simulink model "IBR_Control_2024b"  (R2024b)
settings: Solver=ode4  StartTime=0.0  StopTime=1  FixedStep=Ts  RelTol=1e-3
values from neighbouring files (symbols this model uses):
  Fn = Simulink.Parameter    [IBR_Control_Parameters.m]
  Iang0_pcc = Simulink.Parameter    [IBR_Control_Parameters.m]
  Imag0_pcc = Simulink.Parameter    [IBR_Control_Parameters.m]
  Ki_I = Simulink.Parameter    [IBR_Control_Parameters.m]
  Ki_PLL = Simulink.Parameter    [IBR_Control_Parameters.m]
  Kp_I = Simulink.Parameter    [IBR_Control_Parameters.m]
  Kp_PLL = Simulink.Parameter    [IBR_Control_Parameters.m]
  Lc = Simulink.Parameter    [IBR_Control_Parameters.m]
  Pref = Simulink.Parameter    [IBR_Control_Parameters.m]
  Qref = Simulink.Parameter    [IBR_Control_Parameters.m]
  Rc = Simulink.Parameter    [IBR_Control_Parameters.m]
  Tf_S = Simulink.Parameter    [IBR_Control_Parameters.m]
  Ts = Simulink.Parameter    [IBR_Control_Parameters.m]
  Vang0_pcc = Simulink.Parameter    [IBR_Control_Parameters.m]
  Vmag0_pcc = Simulink.Parameter    [IBR_Control_Parameters.m]
undefined symbols (not defined in the file or in its folder): DiscIntNeverNeededParam
libraries: slpidlib x3, model_info x1
settings Model: ParamWorkspaceSource=ReferencedWorkspace  Creator=evansolingen  LastModifiedBy=if47izeq
settings DataIOCC: LimitDataPoints=on  SaveFormat=Array  SignalLoggingSaveFormat=ModelDataLogs  SaveOutput=off  SignalLogging=off  SaveTime=off  ReturnWorkspaceOutputs=off
settings OptimizationCC: EnhancedBackFolding=on  ExpressionFolding=off  PassReuseOutputArgsThreshold=0  ExpressionDepthLimit=2147483647  OptimizeBlockOrder=speed  DifferentSizesBufferReuse=on
settings DebuggingCC: UnderspecifiedInitializationDetection=Classic  MergeDetectMultiDrivingBlocksExec=none  SolverPrmCheckMsg=warning  MultiTaskDSMMsg=warning  MultiTaskCondExecSysMsg=none  ParameterTunabilityLossMsg=error  FcnCallInpInsideContextMsg=warning  UnconnectedInputMsg=warning  UnconnectedOutputMsg=warning  UnconnectedLineMsg=warning  AllowSymbolicDim=off  StateNameClashWarn=warning  SFUnexpectedBacktrackingDiag=warning  SFNoUnconditionalDefaultTransitionDiag=warning  SFExecutionAtInitializationDiag=none  ArithmeticOperatorsInVariantConditions=warning
settings HardwareCC: ProdBitPerPointer=32  ProdBitPerSizeT=32  ProdBitPerPtrDiffT=32  ProdLargestAtomicFloat=None  ProdIntDivRoundTo=Undefined  ProdEndianess=Unspecified  ProdWordSize=32  ProdHWDeviceType=32-bit Generic
settings ModelReferenceCC: UpdateModelReferenceTargets=Force  EnableRefExpFcnMdlSchedulingChecks=on  PropagateSignalLabelsOutOfModel=off
settings SFSimCC: SimUseLocalCustomCode=off  SimParseCustomCode=off  MATLABDynamicMemAlloc=off  CustomCodeUndefinedFunction=UseInterfaceOnly
settings RTWCC: Description=Create Visual C/C++ Solution File for Simulink Coder  SystemTargetFile=IEC61400_27_DLL.tlc  TemplateMakefile=IEC61400_27_DLL.tmf  RTWUseLocalCustomCode=off  GPUComputeCapability=3.5
settings CodeAppCC: ForceParamTrailComments=on  OperatorAnnotations=on
settings STFCustomTargetCC: ModelReferenceCompliant=off  MATLABClassNameForMDSCustomization=Simulink.SoftwareTarget.TargetSpecificTriggerConfigurationBase  GRTInterface=on  SystemTargetFile=IEC61400_27_DLL.tlc
settings ConfigComp: CovMetricSettings=dw  CovSaveCumulativeToWorkspaceVar=on  CovSaveSingleToWorkspaceVar=on  CovExternalEMLEnable=off

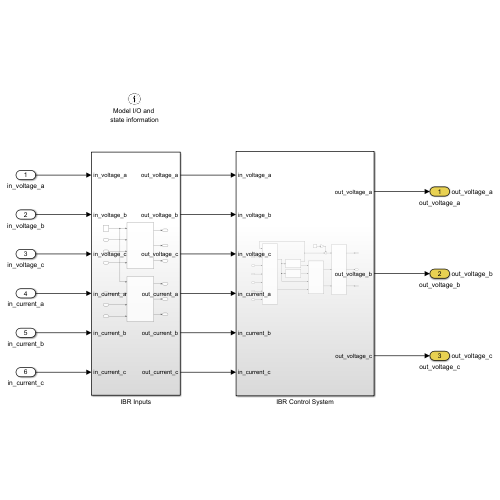
[thumbnail: Simulink's stored preview of the top-level diagram]
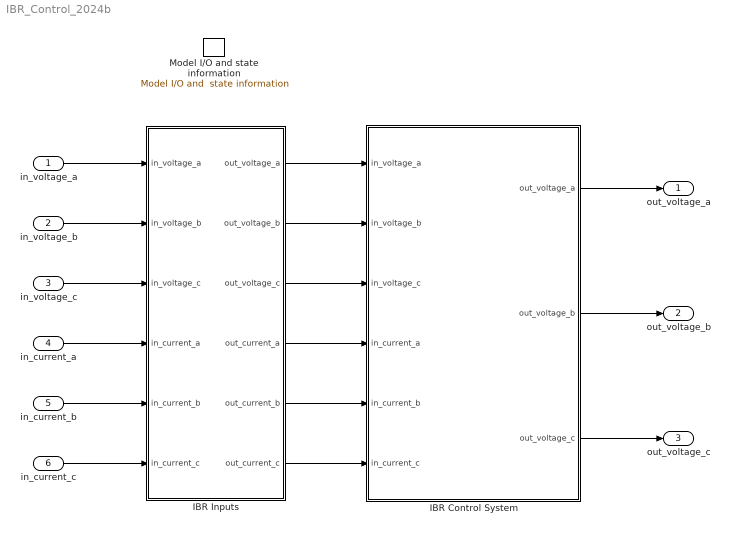
== system IBR_Control_2024b ==
  in_voltage_a : Inport
  in_voltage_b : Inport  Port=2
  in_voltage_c : Inport  Port=3
  in_current_a : Inport  Port=4
  in_current_b : Inport  Port=5
  in_current_c : Inport  Port=6
  IBR Control System : Subsystem
  IBR Inputs : Subsystem
  Model I/O and state information : model_info/Model I//O and  state information
  out_voltage_a : Outport  SignalName=out_voltage_a
  out_voltage_b : Outport  Port=2  SignalName=out_voltage_b
  out_voltage_c : Outport  Port=3  SignalName=out_voltage_c
  wires:
  IBR Control System/1(out_voltage_a) -> out_voltage_a/1
  IBR Control System/2(out_voltage_b) -> out_voltage_b/1
  IBR Control System/3(out_voltage_c) -> out_voltage_c/1
  in_voltage_a/1 -> IBR Inputs/1(in_voltage_a)
  in_voltage_b/1 -> IBR Inputs/2(in_voltage_b)
  in_voltage_c/1 -> IBR Inputs/3(in_voltage_c)
  in_current_a/1 -> IBR Inputs/4(in_current_a)
  in_current_b/1 -> IBR Inputs/5(in_current_b)
  in_current_c/1 -> IBR Inputs/6(in_current_c)
  IBR Inputs/1(out_voltage_a) -> IBR Control System/1(in_voltage_a)
  IBR Inputs/2(out_voltage_b) -> IBR Control System/2(in_voltage_b)
  IBR Inputs/3(out_voltage_c) -> IBR Control System/3(in_voltage_c)
  IBR Inputs/4(out_current_a) -> IBR Control System/4(in_current_a)
  IBR Inputs/6(out_current_c) -> IBR Control System/6(in_current_c)
  IBR Inputs/5(out_current_b) -> IBR Control System/5(in_current_b)

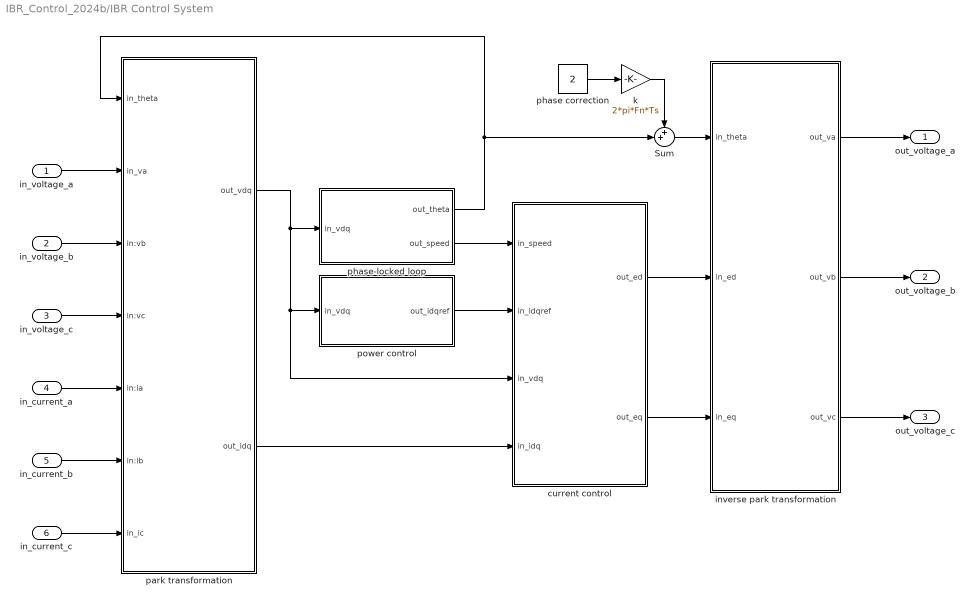
== system IBR_Control_2024b/IBR Control System ==
  in_voltage_a : Inport
  in_voltage_b : Inport  Port=2
  in_voltage_c : Inport  Port=3
  in_current_a : Inport  Port=4
  in_current_b : Inport  Port=5
  in_current_c : Inport  Port=6
  Sum : Sum  Inputs=++|
  current control : Subsystem
  inverse park transformation : Subsystem
  k : Gain  Gain=2*pi*Fn*Ts
  park transformation : Subsystem
  phase correction : Constant  Value=2
  phase-locked loop : Subsystem
  power control : Subsystem
  out_voltage_a : Outport
  out_voltage_b : Outport  Port=2
  out_voltage_c : Outport  Port=3
  wires:
  in_current_b/1 -> park transformation/6(in:ib)
  in_current_c/1 -> park transformation/7(in_ic)
  in_current_a/1 -> park transformation/5(in:ia)
  in_voltage_a/1 -> park transformation/2(in_va)
  in_voltage_b/1 -> park transformation/3(in:vb)
  in_voltage_c/1 -> park transformation/4(in:vc)
  park transformation/1(out_vdq) -> current control/3(in_vdq), power control/1(in_vdq), phase-locked loop/1(in_vdq)
  park transformation/2(out_idq) -> current control/4(in_idq)
  phase-locked loop/2(out_speed) -> current control/1(in_speed)
  power control/1(out_idqref) -> current control/2(in_idqref)
  inverse park transformation/1(out_va) -> out_voltage_a/1
  inverse park transformation/2(out_vb) -> out_voltage_b/1
  inverse park transformation/3(out_vc) -> out_voltage_c/1
  current control/1(out_ed) -> inverse park transformation/2(in_ed)
  current control/2(out_eq) -> inverse park transformation/3(in_eq)
  Sum/1 -> inverse park transformation/1(in_theta)
  phase-locked loop/1(out_theta) -> Sum/2, park transformation/1(in_theta)
  phase correction/1 -> k/1
  k/1 -> Sum/1

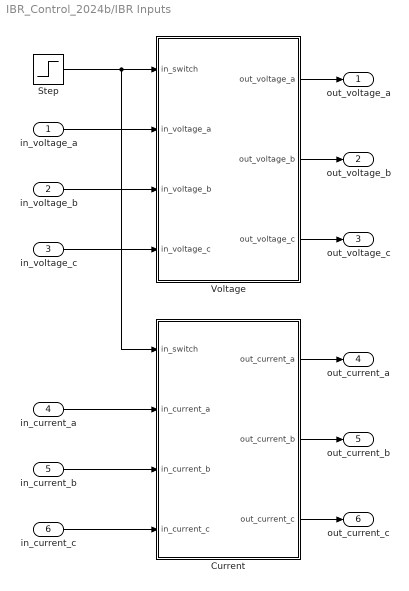
== system IBR_Control_2024b/IBR Inputs ==
  in_voltage_a : Inport
  in_voltage_b : Inport  Port=2
  in_voltage_c : Inport  Port=3
  in_current_a : Inport  Port=4
  in_current_b : Inport  Port=5
  in_current_c : Inport  Port=6
  Current : Subsystem
  Step : Step  Time=3*Ts  Before=1  After=0  SampleTime=0
  Voltage : Subsystem
  out_voltage_a : Outport
  out_voltage_b : Outport  Port=2
  out_voltage_c : Outport  Port=3
  out_current_a : Outport  Port=4
  out_current_b : Outport  Port=5
  out_current_c : Outport  Port=6
  wires:
  Step/1 -> Voltage/1(in_switch), Current/1(in_switch)
  in_voltage_a/1 -> Voltage/2(in_voltage_a)
  in_voltage_c/1 -> Voltage/4(in_voltage_c)
  Voltage/1(out_voltage_a) -> out_voltage_a/1
  Voltage/2(out_voltage_b) -> out_voltage_b/1
  Voltage/3(out_voltage_c) -> out_voltage_c/1
  in_voltage_b/1 -> Voltage/3(in_voltage_b)
  in_current_a/1 -> Current/2(in_current_a)
  in_current_b/1 -> Current/3(in_current_b)
  in_current_c/1 -> Current/4(in_current_c)
  Current/1(out_current_a) -> out_current_a/1
  Current/2(out_current_b) -> out_current_b/1
  Current/3(out_current_c) -> out_current_c/1

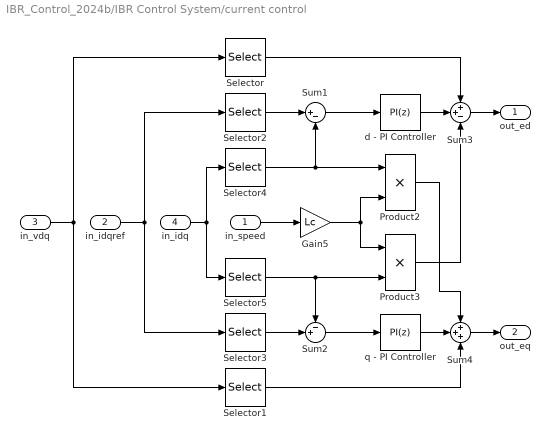
== system IBR_Control_2024b/IBR Control System/current control ==
  in_speed : Inport
  in_idqref : Inport  Port=2
  in_vdq : Inport  Port=3
  in_idq : Inport  Port=4
  Gain5 : Gain  Gain=Lc
  Product2 : Product
  Product3 : Product
  Selector : Selector  InputPortWidth=2  IndexOptions=Index vector (dialog)  Indices=1  OutputSizes=1
  Selector1 : Selector  InputPortWidth=2  IndexOptions=Index vector (dialog)  Indices=[2]  OutputSizes=1
  Selector2 : Selector  InputPortWidth=2  IndexOptions=Index vector (dialog)  Indices=[1]  OutputSizes=1
  Selector3 : Selector  InputPortWidth=2  IndexOptions=Index vector (dialog)  Indices=[2]  OutputSizes=1
  Selector4 : Selector  InputPortWidth=2  IndexOptions=Index vector (dialog)  Indices=[1]  OutputSizes=1
  Selector5 : Selector  InputPortWidth=2  IndexOptions=Index vector (dialog)  Indices=[2]  OutputSizes=1
  Sum1 : Sum  Inputs=|+-
  Sum2 : Sum  Inputs=-+|
  Sum3 : Sum  Inputs=++-
  Sum4 : Sum  Inputs=+++
  d - PI Controller : slpidlib/PID Controller  Controller=PI  Form=Parallel  TimeDomain=Discrete-time  UseExternalTs=off  SampleTime=-1  IntegratorMethod=Forward Euler  FilterMethod=Forward Euler  ControllerParametersSource=internal  P=Kp_I  I=Ki_I  UseKiTs=off  D=0  UseExternalDerivativeSource=off  N=100  UseFilter=on  TunerSelectOption=Transfer Function Based (PID Tuner App)  InitialConditionSource=internal  InitialConditionForIntegrator=Pref/(sqrt(3)/sqrt(2)*Vmag0_pcc)*Rc  InitialConditionForFilter=0  DifferentiatorICPrevScaledInput=0  ExternalReset=none  TrackingMode=off  Kt=1  LimitOutput=off  SatLimitsSource=internal  UpperSaturationLimit=inf  LowerSaturationLimit=-inf  LinearizeAsGain=on  AntiWindupMode=none  Kb=1  LimitIntegrator=off  UpperIntegratorSaturationLimit=inf  LowerIntegratorSaturationLimit=-inf  POutMin=[]  POutMax=[]  IOutMin=[]  IOutMax=[]  DOutMin=[]  DOutMax=[]  NOutMin=[]  NOutMax=[]  SumOutMin=[]  SumOutMax=[]  SaturationOutMin=[]  SaturationOutMax=[]  PParamMin=[]  PParamMax=[]  IParamMin=[]  IParamMax=[]  DParamMin=[]  DParamMax=[]  NParamMin=[]  NParamMax=[]  KbParamMin=[]  KbParamMax=[]  KtParamMin=[]  KtParamMax=[]  KbOutMin=[]  KbOutMax=[]  KtOutMin=[]  KtOutMax=[]  IntegratorOutMin=[]  IntegratorOutMax=[]  FilterOutMin=[]  FilterOutMax=[]  SumI1OutMin=[]  SumI1OutMax=[]  SumI2OutMin=[]  SumI2OutMax=[]  SumI3OutMin=[]  SumI3OutMax=[]  SumI4OutMin=[]  SumI4OutMax=[]  SumDOutMin=[]  SumDOutMax=[]  DifferentiatorOutMin=[]  DifferentiatorOutMax=[]  FilterDiffOutCoefMin=[]  FilterDiffOutCoefMax=[]  ReciprocalOutMin=[]  ReciprocalOutMax=[]  SumDenOutMin=[]  SumDenOutMax=[]  SumNumOutMin=[]  SumNumOutMax=[]  DivideOutMin=[]  DivideOutMax=[]  UdiffTsProdOutMin=[]  UdiffTsProdOutMax=[]  NTsProdOutMin=[]  NTsProdOutMax=[]  UintegralTsProdOutMin=[]  UintegralTsProdOutMax=[]  UngainTsProdOutMin=[]  UngainTsProdOutMax=[]  ClampingZeroOutDataTypeStr=Inherit: Inherit via back propagation  ClampingZeroOutMin=[]  ClampingZeroOutMax=[]  FilterDenConstantOutDataTypeStr=Inherit: Inherit via back propagation  FilterDenConstantOutMin=[]  FilterDenConstantOutMax=[]  PCopyOutDataTypeStr=Inherit: Inherit via back propagation  PCopyOutMin=[]  PCopyOutMax=[]  NCopyOutDataTypeStr=Inherit: Inherit via back propagation  NCopyOutMin=[]  NCopyOutMax=[]  IntegratorContinuousStateAttributes=''  IntegratorStateMustResolveToSignalObject=off  IntegratorRTWStateStorageClass=Auto  FilterContinuousStateAttributes=''  FilterStateMustResolveToSignalObject=off  FilterRTWStateStorageClass=Auto  ParallelPVariant=InternalParameters  IdealPVariant=Disabled  IVariant=InternalParameters  DVariant=Disabled  IntegratorVariant=Discrete  SatVariant=Disabled  AWVariant=Passthrough  PCopyVariant=Disabled  TRVariant=Disabled  FdbkBlocksVariant=Forward  IdealPFdbkVariant=Disabled  SatFdbkVariant=Disabled  DerivativeFilterVariant=Disabled  NVariant=Disabled  NCopyVariant=Disabled_SignalSpec  FilterICVariant=Disabled  IntegratorICVariant=InternalICs  ExternalResetVariant=Disabled  TRSumVariant=Passthrough  SumFdbkVariant=Disabled  SumVariant=Sum_PI  TsampFilterVariant=InternalTs  TsampNgainVariant=Passthrough  TsampIntegralVariant=Disabled_SignalSpec  ExternalSaturationOutDataTypeStr=Inherit: Same as second input  DerivativeSourceVariant=Disabled  PreIntVariant=InternalPreInt
  q - PI Controller : slpidlib/PID Controller  Controller=PI  Form=Parallel  TimeDomain=Discrete-time  UseExternalTs=off  SampleTime=-1  IntegratorMethod=Forward Euler  FilterMethod=Forward Euler  ControllerParametersSource=internal  P=Kp_I  I=Ki_I  UseKiTs=off  D=0  UseExternalDerivativeSource=off  N=100  UseFilter=on  TunerSelectOption=Transfer Function Based (PID Tuner App)  InitialConditionSource=internal  InitialConditionForIntegrator=-Qref/(sqrt(3)/sqrt(2)*Vmag0_pcc)*Rc  InitialConditionForFilter=0  DifferentiatorICPrevScaledInput=0  ExternalReset=none  TrackingMode=off  Kt=1  LimitOutput=off  SatLimitsSource=internal  UpperSaturationLimit=inf  LowerSaturationLimit=-inf  LinearizeAsGain=on  AntiWindupMode=none  Kb=1  LimitIntegrator=off  UpperIntegratorSaturationLimit=inf  LowerIntegratorSaturationLimit=-inf  POutMin=[]  POutMax=[]  IOutMin=[]  IOutMax=[]  DOutMin=[]  DOutMax=[]  NOutMin=[]  NOutMax=[]  SumOutMin=[]  SumOutMax=[]  SaturationOutMin=[]  SaturationOutMax=[]  PParamMin=[]  PParamMax=[]  IParamMin=[]  IParamMax=[]  DParamMin=[]  DParamMax=[]  NParamMin=[]  NParamMax=[]  KbParamMin=[]  KbParamMax=[]  KtParamMin=[]  KtParamMax=[]  KbOutMin=[]  KbOutMax=[]  KtOutMin=[]  KtOutMax=[]  IntegratorOutMin=[]  IntegratorOutMax=[]  FilterOutMin=[]  FilterOutMax=[]  SumI1OutMin=[]  SumI1OutMax=[]  SumI2OutMin=[]  SumI2OutMax=[]  SumI3OutMin=[]  SumI3OutMax=[]  SumI4OutMin=[]  SumI4OutMax=[]  SumDOutMin=[]  SumDOutMax=[]  DifferentiatorOutMin=[]  DifferentiatorOutMax=[]  FilterDiffOutCoefMin=[]  FilterDiffOutCoefMax=[]  ReciprocalOutMin=[]  ReciprocalOutMax=[]  SumDenOutMin=[]  SumDenOutMax=[]  SumNumOutMin=[]  SumNumOutMax=[]  DivideOutMin=[]  DivideOutMax=[]  UdiffTsProdOutMin=[]  UdiffTsProdOutMax=[]  NTsProdOutMin=[]  NTsProdOutMax=[]  UintegralTsProdOutMin=[]  UintegralTsProdOutMax=[]  UngainTsProdOutMin=[]  UngainTsProdOutMax=[]  ClampingZeroOutDataTypeStr=Inherit: Inherit via back propagation  ClampingZeroOutMin=[]  ClampingZeroOutMax=[]  FilterDenConstantOutDataTypeStr=Inherit: Inherit via back propagation  FilterDenConstantOutMin=[]  FilterDenConstantOutMax=[]  PCopyOutDataTypeStr=Inherit: Inherit via back propagation  PCopyOutMin=[]  PCopyOutMax=[]  NCopyOutDataTypeStr=Inherit: Inherit via back propagation  NCopyOutMin=[]  NCopyOutMax=[]  IntegratorContinuousStateAttributes=''  IntegratorStateMustResolveToSignalObject=off  IntegratorRTWStateStorageClass=Auto  FilterContinuousStateAttributes=''  FilterStateMustResolveToSignalObject=off  FilterRTWStateStorageClass=Auto  ParallelPVariant=InternalParameters  IdealPVariant=Disabled  IVariant=InternalParameters  DVariant=Disabled  IntegratorVariant=Discrete  SatVariant=Disabled  AWVariant=Passthrough  PCopyVariant=Disabled  TRVariant=Disabled  FdbkBlocksVariant=Forward  IdealPFdbkVariant=Disabled  SatFdbkVariant=Disabled  DerivativeFilterVariant=Disabled  NVariant=Disabled  NCopyVariant=Disabled_SignalSpec  FilterICVariant=Disabled  IntegratorICVariant=InternalICs  ExternalResetVariant=Disabled  TRSumVariant=Passthrough  SumFdbkVariant=Disabled  SumVariant=Sum_PI  TsampFilterVariant=InternalTs  TsampNgainVariant=Passthrough  TsampIntegralVariant=Disabled_SignalSpec  ExternalSaturationOutDataTypeStr=Inherit: Same as second input  DerivativeSourceVariant=Disabled  PreIntVariant=InternalPreInt
  out_ed : Outport
  out_eq : Outport  Port=2
  wires:
  Gain5/1 -> Product2/2, Product3/1
  Sum4/1 -> out_eq/1
  Product3/1 -> Sum3/3
  Selector3/1 -> Sum2/2
  Sum1/1 -> d - PI Controller/1
  Sum3/1 -> out_ed/1
  Product2/1 -> Sum4/1
  Sum2/1 -> q - PI Controller/1
  in_speed/1 -> Gain5/1
  in_vdq/1 -> Selector1/1, Selector/1
  in_idq/1 -> Selector5/1, Selector4/1
  Selector5/1 -> Product3/2, Sum2/1
  d - PI Controller/1 -> Sum3/2
  q - PI Controller/1 -> Sum4/2
  Selector1/1 -> Sum4/3
  in_idqref/1 -> Selector2/1, Selector3/1
  Selector2/1 -> Sum1/1
  Selector/1 -> Sum3/1
  Selector4/1 -> Product2/1, Sum1/2

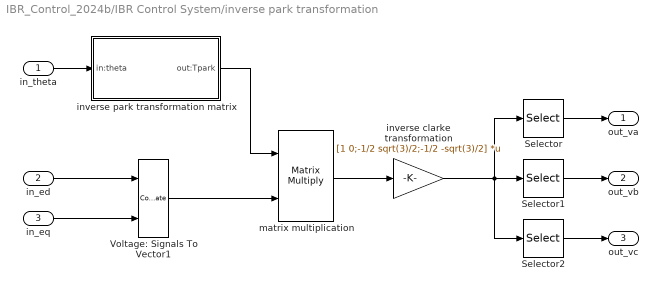
== system IBR_Control_2024b/IBR Control System/inverse park transformation ==
  in_theta : Inport
  in_ed : Inport  Port=2
  in_eq : Inport  Port=3
  Selector : Selector  InputPortWidth=3  IndexOptions=Index vector (dialog)  Indices=[1]  OutputSizes=1
  Selector1 : Selector  InputPortWidth=3  IndexOptions=Index vector (dialog)  Indices=[2]  OutputSizes=1
  Selector2 : Selector  InputPortWidth=3  IndexOptions=Index vector (dialog)  Indices=[3]  OutputSizes=1
  Voltage: Signals To Vector1 : Concatenate  Mode=Multidimensional array
  inverse clarke transformation : Gain  Gain=[1 0;-1/2 sqrt(3)/2;-1/2 -sqrt(3)/2]  Multiplication=Matrix(K*u)
  inverse park transformation matrix : Subsystem
  matrix multiplication : Product  Multiplication=Matrix(*)
  out_va : Outport
  out_vb : Outport  Port=2
  out_vc : Outport  Port=3
  wires:
  inverse park transformation matrix/1(out:Tpark) -> matrix multiplication/1
  in_theta/1 -> inverse park transformation matrix/1(in:theta)
  inverse clarke transformation/1 -> Selector2/1, Selector1/1, Selector/1
  matrix multiplication/1 -> inverse clarke transformation/1
  Selector1/1 -> out_vb/1
  Selector/1 -> out_va/1
  in_ed/1 -> Voltage: Signals To Vector1/1
  in_eq/1 -> Voltage: Signals To Vector1/2
  Voltage: Signals To Vector1/1 -> matrix multiplication/2
  Selector2/1 -> out_vc/1

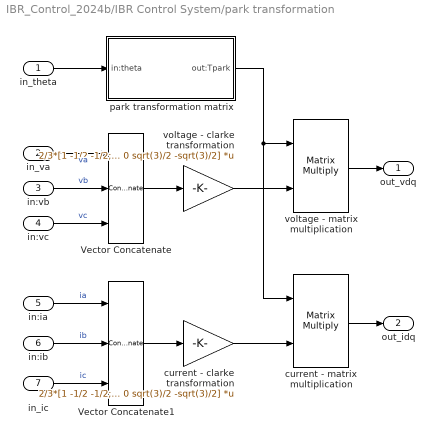
== system IBR_Control_2024b/IBR Control System/park transformation ==
  in_theta : Inport
  in_va : Inport  Port=2
  in:vb : Inport  Port=3
  in:vc : Inport  Port=4
  in:ia : Inport  Port=5
  in:ib : Inport  Port=6
  in_ic : Inport  Port=7
  Vector Concatenate : Concatenate  NumInputs=3  Mode=Multidimensional array
  Vector Concatenate1 : Concatenate  NumInputs=3  Mode=Multidimensional array
  current - clarke transformation : Gain  Gain=2/3*[1 -1/2 -1/2; 0 sqrt(3)/2 -sqrt(3)/2]  Multiplication=Matrix(K*u)
  current - matrix multiplication : Product  Multiplication=Matrix(*)
  park transformation matrix : Subsystem
  voltage - clarke transformation : Gain  Gain=2/3*[1 -1/2 -1/2; 0 sqrt(3)/2 -sqrt(3)/2]  Multiplication=Matrix(K*u)
  voltage - matrix multiplication : Product  Multiplication=Matrix(*)
  out_vdq : Outport
  out_idq : Outport  Port=2
  wires:
  in_va/1 -> Vector Concatenate/1  "va"
  in:ib/1 -> Vector Concatenate1/2  "ib"
  in_ic/1 -> Vector Concatenate1/3  "ic"
  Vector Concatenate1/1 -> current - clarke transformation/1
  in:ia/1 -> Vector Concatenate1/1  "ia"
  voltage - matrix multiplication/1 -> out_vdq/1
  in:vb/1 -> Vector Concatenate/2  "vb"
  in:vc/1 -> Vector Concatenate/3  "vc"
  Vector Concatenate/1 -> voltage - clarke transformation/1
  voltage - clarke transformation/1 -> voltage - matrix multiplication/2
  current - clarke transformation/1 -> current - matrix multiplication/2
  park transformation matrix/1(out:Tpark) -> voltage - matrix multiplication/1, current - matrix multiplication/1
  current - matrix multiplication/1 -> out_idq/1
  in_theta/1 -> park transformation matrix/1(in:theta)

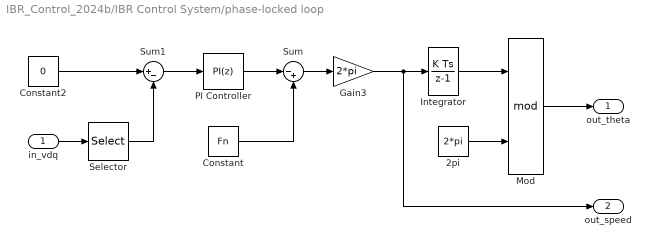
== system IBR_Control_2024b/IBR Control System/phase-locked loop ==
  in_vdq : Inport
  2pi : Constant  Value=2*pi
  Constant : Constant  Value=Fn
  Constant2 : Constant  Value=0
  Gain3 : Gain  Gain=2*pi
  Integrator : DiscreteIntegrator  InitialCondition=Vang0_pcc-2*2*pi*Fn*Ts  SampleTime=-1  ICPrevOutput=DiscIntNeverNeededParam  ICPrevScaledInput=DiscIntNeverNeededParam
  Mod : Math  Operator=mod
  PI Controller : slpidlib/PID Controller  Controller=PI  Form=Parallel  TimeDomain=Discrete-time  UseExternalTs=off  SampleTime=-1  IntegratorMethod=Forward Euler  FilterMethod=Forward Euler  ControllerParametersSource=internal  P=Kp_PLL  I=Ki_PLL  UseKiTs=off  D=0  UseExternalDerivativeSource=off  N=100  UseFilter=on  TunerSelectOption=Transfer Function Based (PID Tuner App)  InitialConditionSource=internal  InitialConditionForIntegrator=0  InitialConditionForFilter=0  DifferentiatorICPrevScaledInput=0  ExternalReset=none  TrackingMode=off  Kt=1  LimitOutput=off  SatLimitsSource=internal  UpperSaturationLimit=inf  LowerSaturationLimit=-inf  LinearizeAsGain=on  AntiWindupMode=none  Kb=1  LimitIntegrator=off  UpperIntegratorSaturationLimit=inf  LowerIntegratorSaturationLimit=-inf  POutMin=[]  POutMax=[]  IOutMin=[]  IOutMax=[]  DOutMin=[]  DOutMax=[]  NOutMin=[]  NOutMax=[]  SumOutMin=[]  SumOutMax=[]  SaturationOutMin=[]  SaturationOutMax=[]  PParamMin=[]  PParamMax=[]  IParamMin=[]  IParamMax=[]  DParamMin=[]  DParamMax=[]  NParamMin=[]  NParamMax=[]  KbParamMin=[]  KbParamMax=[]  KtParamMin=[]  KtParamMax=[]  KbOutMin=[]  KbOutMax=[]  KtOutMin=[]  KtOutMax=[]  IntegratorOutMin=[]  IntegratorOutMax=[]  FilterOutMin=[]  FilterOutMax=[]  SumI1OutMin=[]  SumI1OutMax=[]  SumI2OutMin=[]  SumI2OutMax=[]  SumI3OutMin=[]  SumI3OutMax=[]  SumI4OutMin=[]  SumI4OutMax=[]  SumDOutMin=[]  SumDOutMax=[]  DifferentiatorOutMin=[]  DifferentiatorOutMax=[]  FilterDiffOutCoefMin=[]  FilterDiffOutCoefMax=[]  ReciprocalOutMin=[]  ReciprocalOutMax=[]  SumDenOutMin=[]  SumDenOutMax=[]  SumNumOutMin=[]  SumNumOutMax=[]  DivideOutMin=[]  DivideOutMax=[]  UdiffTsProdOutMin=[]  UdiffTsProdOutMax=[]  NTsProdOutMin=[]  NTsProdOutMax=[]  UintegralTsProdOutMin=[]  UintegralTsProdOutMax=[]  UngainTsProdOutMin=[]  UngainTsProdOutMax=[]  ClampingZeroOutDataTypeStr=Inherit: Inherit via back propagation  ClampingZeroOutMin=[]  ClampingZeroOutMax=[]  FilterDenConstantOutDataTypeStr=Inherit: Inherit via back propagation  FilterDenConstantOutMin=[]  FilterDenConstantOutMax=[]  PCopyOutDataTypeStr=Inherit: Inherit via back propagation  PCopyOutMin=[]  PCopyOutMax=[]  NCopyOutDataTypeStr=Inherit: Inherit via back propagation  NCopyOutMin=[]  NCopyOutMax=[]  IntegratorContinuousStateAttributes=''  IntegratorStateMustResolveToSignalObject=off  IntegratorRTWStateStorageClass=Auto  FilterContinuousStateAttributes=''  FilterStateMustResolveToSignalObject=off  FilterRTWStateStorageClass=Auto  ParallelPVariant=InternalParameters  IdealPVariant=Disabled  IVariant=InternalParameters  DVariant=Disabled  IntegratorVariant=Discrete  SatVariant=Disabled  AWVariant=Passthrough  PCopyVariant=Disabled  TRVariant=Disabled  FdbkBlocksVariant=Forward  IdealPFdbkVariant=Disabled  SatFdbkVariant=Disabled  DerivativeFilterVariant=Disabled  NVariant=Disabled  NCopyVariant=Disabled_SignalSpec  FilterICVariant=Disabled  IntegratorICVariant=InternalICs  ExternalResetVariant=Disabled  TRSumVariant=Passthrough  SumFdbkVariant=Disabled  SumVariant=Sum_PI  TsampFilterVariant=InternalTs  TsampNgainVariant=Passthrough  TsampIntegralVariant=Disabled_SignalSpec  ExternalSaturationOutDataTypeStr=Inherit: Same as second input  DerivativeSourceVariant=Disabled  PreIntVariant=InternalPreInt
  Selector : Selector  InputPortWidth=2  IndexOptions=Index vector (dialog)  Indices=[2]  OutputSizes=1
  Sum : Sum  Inputs=|-+
  Sum1 : Sum  Inputs=|+-
  out_theta : Outport
  out_speed : Outport  Port=2
  wires:
  Constant/1 -> Sum/2
  Sum/1 -> Gain3/1
  2pi/1 -> Mod/2
  Gain3/1 -> out_speed/1, Integrator/1
  Sum1/1 -> PI Controller/1
  Mod/1 -> out_theta/1
  in_vdq/1 -> Selector/1
  Selector/1 -> Sum1/2
  Constant2/1 -> Sum1/1
  PI Controller/1 -> Sum/1
  Integrator/1 -> Mod/1

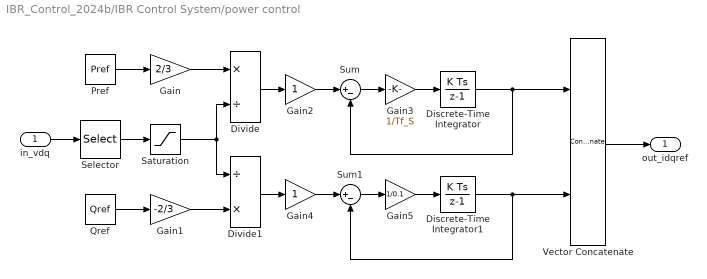
== system IBR_Control_2024b/IBR Control System/power control ==
  in_vdq : Inport
  Discrete-Time Integrator : DiscreteIntegrator  InitialCondition=Pref/(sqrt(3)/sqrt(2)*Vmag0_pcc)  SampleTime=-1  ICPrevOutput=DiscIntNeverNeededParam  ICPrevScaledInput=DiscIntNeverNeededParam
  Discrete-Time Integrator1 : DiscreteIntegrator  InitialCondition=-Qref/(sqrt(3)/sqrt(2)*Vmag0_pcc)  SampleTime=-1  ICPrevOutput=DiscIntNeverNeededParam  ICPrevScaledInput=DiscIntNeverNeededParam
  Divide : Product  Inputs=*/
  Divide1 : Product  Inputs=/*
  Gain : Gain  Gain=2/3
  Gain1 : Gain  Gain=-2/3
  Gain2 : Gain
  Gain3 : Gain  Gain=1/Tf_S
  Gain4 : Gain
  Gain5 : Gain  Gain=1/0.1
  Pref : Constant  Value=Pref
  Qref : Constant  Value=Qref
  Saturation : Saturate  UpperLimit=inf  LowerLimit=0.1
  Selector : Selector  InputPortWidth=2  IndexOptions=Index vector (dialog)  Indices=[1]  OutputSizes=1
  Sum : Sum  Inputs=|+-
  Sum1 : Sum  Inputs=|+-
  Vector Concatenate : Concatenate  Mode=Multidimensional array
  out_idqref : Outport
  wires:
  Pref/1 -> Gain/1
  Gain/1 -> Divide/1
  Qref/1 -> Gain1/1
  Selector/1 -> Saturation/1
  Gain1/1 -> Divide1/2
  in_vdq/1 -> Selector/1
  Vector Concatenate/1 -> out_idqref/1
  Divide/1 -> Gain2/1
  Gain2/1 -> Sum/1
  Sum/1 -> Gain3/1
  Gain3/1 -> Discrete-Time Integrator/1
  Discrete-Time Integrator/1 -> Sum/2, Vector Concatenate/1
  Sum1/1 -> Gain5/1
  Gain4/1 -> Sum1/1
  Gain5/1 -> Discrete-Time Integrator1/1
  Discrete-Time Integrator1/1 -> Vector Concatenate/2, Sum1/2
  Divide1/1 -> Gain4/1
  Saturation/1 -> Divide/2, Divide1/1

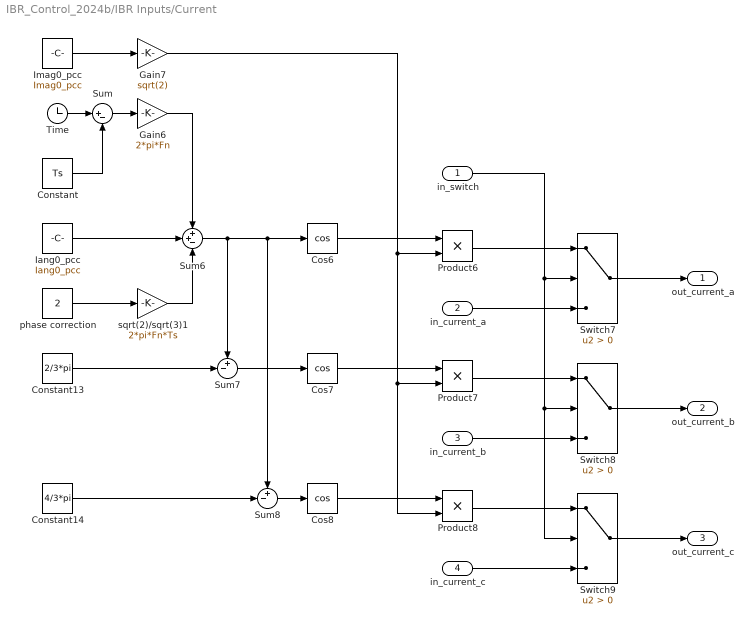
== system IBR_Control_2024b/IBR Inputs/Current ==
  in_switch : Inport
  in_current_a : Inport  Port=2
  in_current_b : Inport  Port=3
  in_current_c : Inport  Port=4
  Constant : Constant  Value=Ts
  Constant13 : Constant  Value=2/3*pi
  Constant14 : Constant  Value=4/3*pi
  Cos6 : Trigonometry  Operator=cos
  Cos7 : Trigonometry  Operator=cos
  Cos8 : Trigonometry  Operator=cos
  Gain6 : Gain  Gain=2*pi*Fn
  Gain7 : Gain  Gain=sqrt(2)
  Iang0_pcc : Constant  Value=Iang0_pcc
  Imag0_pcc : Constant  Value=Imag0_pcc
  Product6 : Product
  Product7 : Product
  Product8 : Product
  Sum : Sum  Inputs=|+-
  Sum6 : Sum  Inputs=++-
  Sum7 : Sum  Inputs=+-|
  Sum8 : Sum  Inputs=+-|
  Switch7 : Switch  Criteria=u2 > Threshold  SaturateOnIntegerOverflow=off  InputSameDT=off
  Switch8 : Switch  Criteria=u2 > Threshold  SaturateOnIntegerOverflow=off  InputSameDT=off
  Switch9 : Switch  Criteria=u2 > Threshold  SaturateOnIntegerOverflow=off  InputSameDT=off
  Time : Clock
  phase correction : Constant  Value=2
  sqrt(2)/sqrt(3)1 : Gain  Gain=2*pi*Fn*Ts
  out_current_a : Outport
  out_current_b : Outport  Port=2
  out_current_c : Outport  Port=3
  wires:
  Sum8/1 -> Cos8/1
  Gain7/1 -> Product8/2, Product7/2, Product6/2
  Cos7/1 -> Product7/1
  Switch9/1 -> out_current_c/1
  Constant14/1 -> Sum8/2
  Sum6/1 -> Cos6/1, Sum8/1, Sum7/1
  in_switch/1 -> Switch8/2, Switch9/2, Switch7/2
  Cos8/1 -> Product8/1
  Cos6/1 -> Product6/1
  Switch7/1 -> out_current_a/1
  Sum7/1 -> Cos7/1
  Iang0_pcc/1 -> Sum6/2
  Imag0_pcc/1 -> Gain7/1
  Product6/1 -> Switch7/1
  in_current_a/1 -> Switch7/3
  in_current_c/1 -> Switch9/3
  Product8/1 -> Switch9/1
  Product7/1 -> Switch8/1
  Constant13/1 -> Sum7/2
  Time/1 -> Sum/1
  Switch8/1 -> out_current_b/1
  in_current_b/1 -> Switch8/3
  phase correction/1 -> sqrt(2)/sqrt(3)1/1
  Gain6/1 -> Sum6/1
  sqrt(2)/sqrt(3)1/1 -> Sum6/3
  Constant/1 -> Sum/2
  Sum/1 -> Gain6/1

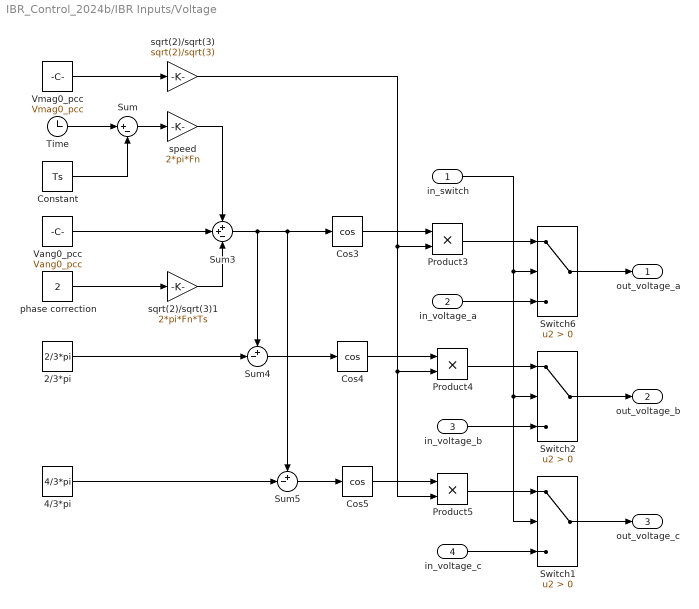
== system IBR_Control_2024b/IBR Inputs/Voltage ==
  in_switch : Inport
  in_voltage_a : Inport  Port=2
  in_voltage_b : Inport  Port=3
  in_voltage_c : Inport  Port=4
  2/3*pi : Constant  Value=2/3*pi
  4/3*pi : Constant  Value=4/3*pi
  Constant : Constant  Value=Ts
  Cos3 : Trigonometry  Operator=cos
  Cos4 : Trigonometry  Operator=cos
  Cos5 : Trigonometry  Operator=cos
  Product3 : Product
  Product4 : Product
  Product5 : Product
  Sum : Sum  Inputs=|+-
  Sum3 : Sum  Inputs=++-
  Sum4 : Sum  Inputs=+-|
  Sum5 : Sum  Inputs=+-|
  Switch1 : Switch  Criteria=u2 > Threshold  SaturateOnIntegerOverflow=off  InputSameDT=off
  Switch2 : Switch  Criteria=u2 > Threshold  SaturateOnIntegerOverflow=off  InputSameDT=off
  Switch6 : Switch  Criteria=u2 > Threshold  SaturateOnIntegerOverflow=off  InputSameDT=off
  Time : Clock
  Vang0_pcc : Constant  Value=Vang0_pcc
  Vmag0_pcc : Constant  Value=Vmag0_pcc
  phase correction : Constant  Value=2
  speed : Gain  Gain=2*pi*Fn
  sqrt(2)/sqrt(3) : Gain  Gain=sqrt(2)/sqrt(3)
  sqrt(2)/sqrt(3)1 : Gain  Gain=2*pi*Fn*Ts
  out_voltage_a : Outport
  out_voltage_b : Outport  Port=2
  out_voltage_c : Outport  Port=3
  wires:
  Vmag0_pcc/1 -> sqrt(2)/sqrt(3)/1
  Sum3/1 -> Sum5/1, Cos3/1, Sum4/1
  in_voltage_c/1 -> Switch1/3
  Sum4/1 -> Cos4/1
  Cos3/1 -> Product3/1
  Switch1/1 -> out_voltage_c/1
  2/3*pi/1 -> Sum4/2
  in_switch/1 -> Switch1/2, Switch2/2, Switch6/2
  Cos5/1 -> Product5/1
  Sum5/1 -> Cos5/1
  phase correction/1 -> sqrt(2)/sqrt(3)1/1
  Product3/1 -> Switch6/1
  Switch6/1 -> out_voltage_a/1
  sqrt(2)/sqrt(3)/1 -> Product5/2, Product4/2, Product3/2
  in_voltage_b/1 -> Switch2/3
  4/3*pi/1 -> Sum5/2
  speed/1 -> Sum3/1
  Product5/1 -> Switch1/1
  Time/1 -> Sum/1
  Product4/1 -> Switch2/1
  Vang0_pcc/1 -> Sum3/2
  Cos4/1 -> Product4/1
  in_voltage_a/1 -> Switch6/3
  Switch2/1 -> out_voltage_b/1
  sqrt(2)/sqrt(3)1/1 -> Sum3/3
  Constant/1 -> Sum/2
  Sum/1 -> speed/1

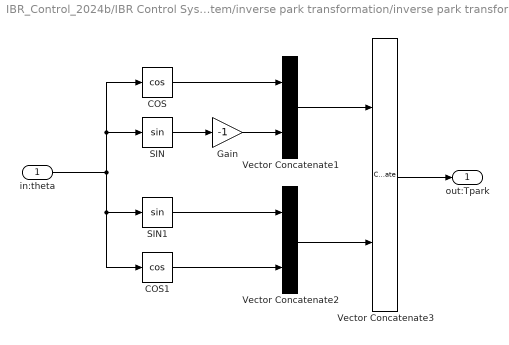
== system IBR_Control_2024b/IBR Control System/inverse park transformation/inverse park transformation matrix ==
  in:theta : Inport
  COS : Trigonometry  Operator=cos
  COS1 : Trigonometry  Operator=cos
  Gain : Gain  Gain=-1
  SIN : Trigonometry
  SIN1 : Trigonometry
  Vector Concatenate1 : Concatenate  Mode=Multidimensional array  ConcatenateDimension=2
  Vector Concatenate2 : Concatenate  Mode=Multidimensional array  ConcatenateDimension=2
  Vector Concatenate3 : Concatenate  Mode=Multidimensional array
  out:Tpark : Outport
  wires:
  Vector Concatenate2/1 -> Vector Concatenate3/2
  COS/1 -> Vector Concatenate1/1
  in:theta/1 -> COS1/1, SIN1/1, COS/1, SIN/1
  SIN/1 -> Gain/1
  Vector Concatenate1/1 -> Vector Concatenate3/1
  SIN1/1 -> Vector Concatenate2/1
  Vector Concatenate3/1 -> out:Tpark/1
  COS1/1 -> Vector Concatenate2/2
  Gain/1 -> Vector Concatenate1/2

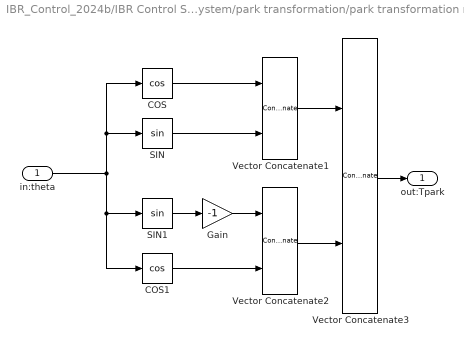
== system IBR_Control_2024b/IBR Control System/park transformation/park transformation matrix ==
  in:theta : Inport
  COS : Trigonometry  Operator=cos
  COS1 : Trigonometry  Operator=cos
  Gain : Gain  Gain=-1
  SIN : Trigonometry
  SIN1 : Trigonometry
  Vector Concatenate1 : Concatenate  Mode=Multidimensional array  ConcatenateDimension=2
  Vector Concatenate2 : Concatenate  Mode=Multidimensional array  ConcatenateDimension=2
  Vector Concatenate3 : Concatenate  Mode=Multidimensional array
  out:Tpark : Outport
  wires:
  Vector Concatenate2/1 -> Vector Concatenate3/2
  COS/1 -> Vector Concatenate1/1
  in:theta/1 -> COS1/1, SIN1/1, COS/1, SIN/1
  SIN/1 -> Vector Concatenate1/2
  Vector Concatenate1/1 -> Vector Concatenate3/1
  Gain/1 -> Vector Concatenate2/1
  Vector Concatenate3/1 -> out:Tpark/1
  SIN1/1 -> Gain/1
  COS1/1 -> Vector Concatenate2/2
